simulink model "AircraftGainScheduling"  (R2022a)
settings: Solver=VariableStepAuto  StartTime=0.0  StopTime=100  RelTol=1e-3
values from neighbouring files (symbols this model uses):
  Amd = (eye(9)+Ts*Am)    [ControlMinimal.m]    (also in ExtendedControl.m; newSys.m)
  Bmd = Ts*Bm    [ControlMinimal.m]    (also in ExtendedControl.m; newSys.m)
  Cm = eye(9)    [newSys.m]
  Cmd = Cm    [ControlMinimal.m]    (also in ExtendedControl.m; newSys.m)
  Kmd = dlqr(Amd,Bmd,Q,R)    [ControlMinimal.m]    (also in ExtendedControl.m; newSys.m = lqr(Am-Ld*Cmd,Bm,Q,R))
  pointOfEquilibrium = PointOfEquilibrium(operationStates, operatingInputs )    [ControllerAroundPointOfOperation.m]    (also in InitializeAircraftPlacePolesCalculateN.m = PointOfEquilibrium([u0;v0;w0;0;0;0;0;Theta0;Psi0;0;0;100].',; TestMergeFinalLoad.m = PointOfEquilibrium(states,inputs,[-1,-1,-1]); extindere_stari_cu_perturbatie.m = PointOfEquilibrium([u0;0;w0;0;0;0;0;Theta0;Psi0;0;0;100].', ; newSys.m = PointOfEquilibrium(operationStates.', operatingInputs ))
  Ts = 0.1    [ControlMinimal.m]    (also in EstimareIntrareNecunoscuta.m; ExtendedControl.m; KalmanFilterForExtendedLinearSystem.m; LoadmUltiplePoint.m)
libraries: sharedtransform x2
settings Model: Creator=Bogdan  LastModifiedBy=Bogdan

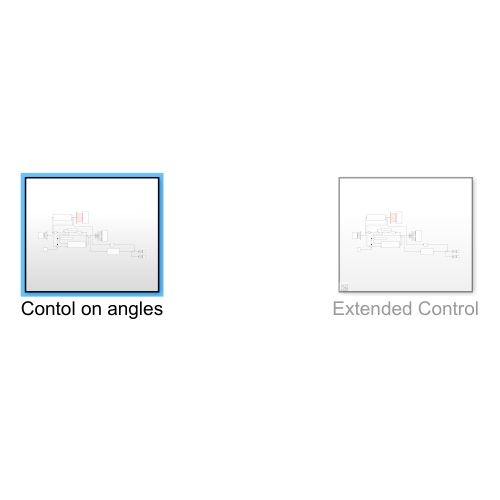
[thumbnail: Simulink's stored preview of the top-level diagram]
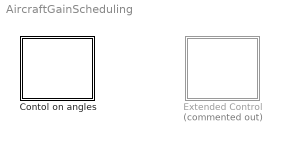
== system AircraftGainScheduling ==
  Contol on angles : Subsystem
  Extended Control : Subsystem  Commented=on

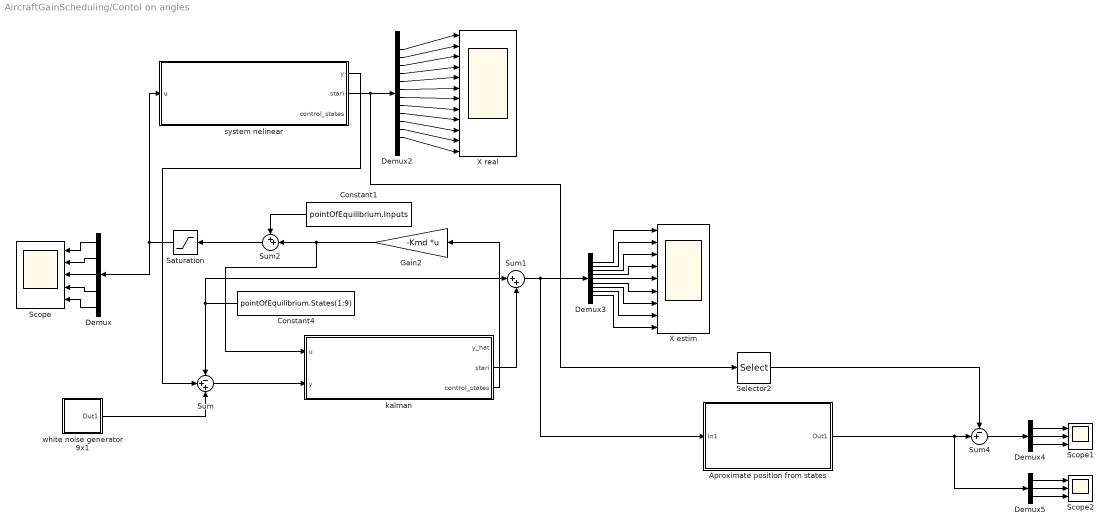
== system AircraftGainScheduling/Contol on angles ==
  Aproximate position from states : Subsystem
  Constant1 : Constant  Value=pointOfEquilibrium.Inputs
  Constant4 : Constant  Value=pointOfEquilibrium.States(1:9)
  Demux : Demux  Outputs=5
  Demux2 : Demux  Outputs=12
  Demux3 : Demux  Outputs=9
  Demux4 : Demux  Outputs=3
  Demux5 : Demux  Outputs=3
  Gain2 : Gain  Gain=-Kmd  Multiplication=Matrix(K*u) (u vector)
  Saturation : Saturate  UpperLimit=[10,pi/6,pi/6,pi/6,pi/6]  LowerLimit=[0,-pi/6,-pi/6,-pi/6,-pi/6]
  Scope : Scope  NumInputPorts=5
  Scope1 : Scope  NumInputPorts=3
  Scope2 : Scope  NumInputPorts=3
  Selector2 : Selector  InputPortWidth=12  IndexOptions=Index vector (dialog)  Indices=[10:12]  OutputSizes=1
  Sum : Sum  Inputs=-++
  Sum1 : Sum  Inputs=|++
  Sum2 : Sum  Inputs=++|
  Sum4 : Sum  Inputs=-+|
  X estim : Scope  NumInputPorts=9
  X real : Scope  NumInputPorts=12
  kalman : Subsystem
  system nelinear : Subsystem
  white noise generator 9x1 : Subsystem
  wires:
  Demux5/2 -> Scope2/2
  Demux/2 -> Scope/2
  Demux2/2 -> X real/2
  Demux3/1 -> X estim/1
  Demux5/3 -> Scope2/3
  system nelinear/2(stari) -> Selector2/1, Demux2/1
  Demux4/2 -> Scope1/2
  Constant4/1 -> Sum1/1, Sum/1
  Demux2/1 -> X real/1
  Demux3/7 -> X estim/7
  Aproximate position from states/1(Out1) -> Demux5/1, Sum4/2
  Demux/1 -> Scope/1
  Demux2/8 -> X real/8
  Demux/3 -> Scope/3
  Demux2/5 -> X real/5
  Demux4/1 -> Scope1/1
  Demux/4 -> Scope/4
  Saturation/1 -> system nelinear/1(u), Demux/1
  kalman/3(control_states) -> Gain2/1
  Demux3/5 -> X estim/5
  Sum2/1 -> Saturation/1
  Demux3/6 -> X estim/6
  Demux2/3 -> X real/3
  Sum/1 -> kalman/2(y)
  Sum1/1 -> Aproximate position from states/1(In1), Demux3/1
  Demux3/8 -> X estim/8
  Demux2/6 -> X real/6
  Sum4/1 -> Demux4/1
  Demux3/4 -> X estim/4
  white noise generator 9x1/1(Out1) -> Sum/3
  Demux5/1 -> Scope2/1
  Demux2/7 -> X real/7
  Demux4/3 -> Scope1/3
  Selector2/1 -> Sum4/1
  Demux3/9 -> X estim/9
  Demux2/11 -> X real/11
  Constant1/1 -> Sum2/1
  Demux2/12 -> X real/12
  Demux2/10 -> X real/10
  kalman/2(stari) -> Sum1/2
  Gain2/1 -> Sum2/2, kalman/1(u)
  Demux3/3 -> X estim/3
  Demux2/4 -> X real/4
  Demux3/2 -> X estim/2
  Demux/5 -> Scope/5
  Demux2/9 -> X real/9
  system nelinear/1(y) -> Sum/2

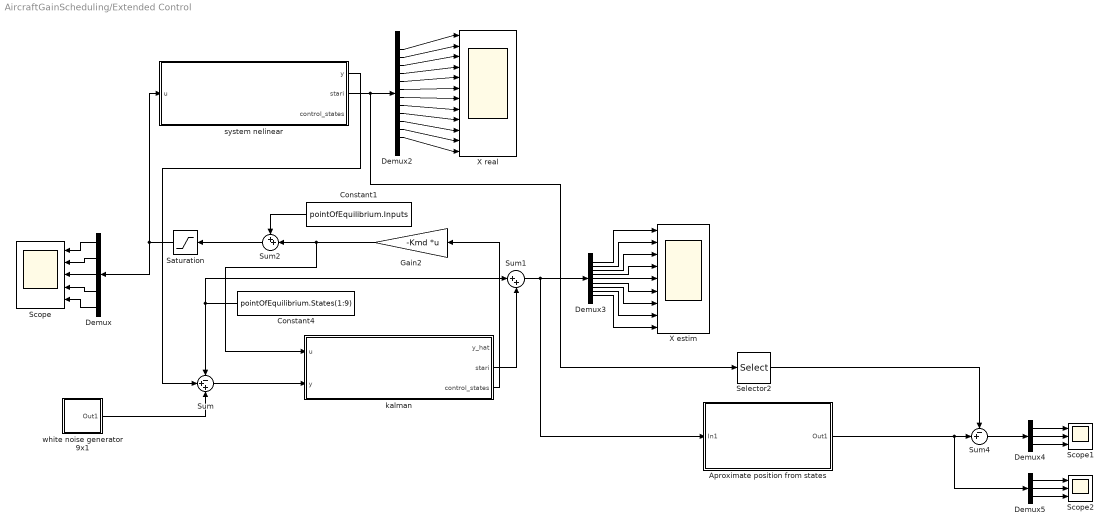
== system AircraftGainScheduling/Extended Control ==
  Aproximate position from states : Subsystem
  Constant1 : Constant  Value=pointOfEquilibrium.Inputs
  Constant4 : Constant  Value=pointOfEquilibrium.States(1:9)
  Demux : Demux  Outputs=5
  Demux2 : Demux  Outputs=12
  Demux3 : Demux  Outputs=9
  Demux4 : Demux  Outputs=3
  Demux5 : Demux  Outputs=3
  Gain2 : Gain  Gain=-Kmd  Multiplication=Matrix(K*u) (u vector)
  Saturation : Saturate  UpperLimit=[10,pi/6,pi/6,pi/6,pi/6]  LowerLimit=[0,-pi/6,-pi/6,-pi/6,-pi/6]
  Scope : Scope  NumInputPorts=5
  Scope1 : Scope  NumInputPorts=3
  Scope2 : Scope  NumInputPorts=3
  Selector2 : Selector  InputPortWidth=12  IndexOptions=Index vector (dialog)  Indices=[10:12]  OutputSizes=1
  Sum : Sum  Inputs=-++
  Sum1 : Sum  Inputs=|++
  Sum2 : Sum  Inputs=++|
  Sum4 : Sum  Inputs=-+|
  X estim : Scope  NumInputPorts=9
  X real : Scope  NumInputPorts=12
  kalman : Subsystem
  system nelinear : Subsystem
  white noise generator 9x1 : Subsystem
  wires:
  Demux5/2 -> Scope2/2
  Demux/2 -> Scope/2
  Demux2/2 -> X real/2
  Demux3/1 -> X estim/1
  Demux5/3 -> Scope2/3
  system nelinear/2(stari) -> Selector2/1, Demux2/1
  Demux4/2 -> Scope1/2
  Constant4/1 -> Sum1/1, Sum/1
  Demux2/1 -> X real/1
  Demux3/7 -> X estim/7
  Aproximate position from states/1(Out1) -> Demux5/1, Sum4/2
  Demux/1 -> Scope/1
  Demux2/8 -> X real/8
  Demux/3 -> Scope/3
  Demux2/5 -> X real/5
  Demux4/1 -> Scope1/1
  Demux/4 -> Scope/4
  Saturation/1 -> system nelinear/1(u), Demux/1
  kalman/3(control_states) -> Gain2/1
  Demux3/5 -> X estim/5
  Sum2/1 -> Saturation/1
  Demux3/6 -> X estim/6
  Demux2/3 -> X real/3
  Sum/1 -> kalman/2(y)
  Sum1/1 -> Aproximate position from states/1(In1), Demux3/1
  Demux3/8 -> X estim/8
  Demux2/6 -> X real/6
  Sum4/1 -> Demux4/1
  Demux3/4 -> X estim/4
  white noise generator 9x1/1(Out1) -> Sum/3
  Demux5/1 -> Scope2/1
  Demux2/7 -> X real/7
  Demux4/3 -> Scope1/3
  Selector2/1 -> Sum4/1
  Demux3/9 -> X estim/9
  Demux2/11 -> X real/11
  Constant1/1 -> Sum2/1
  Demux2/12 -> X real/12
  Demux2/10 -> X real/10
  kalman/2(stari) -> Sum1/2
  Gain2/1 -> Sum2/2, kalman/1(u)
  Demux3/3 -> X estim/3
  Demux2/4 -> X real/4
  Demux3/2 -> X estim/2
  Demux/5 -> Scope/5
  Demux2/9 -> X real/9
  system nelinear/1(y) -> Sum/2

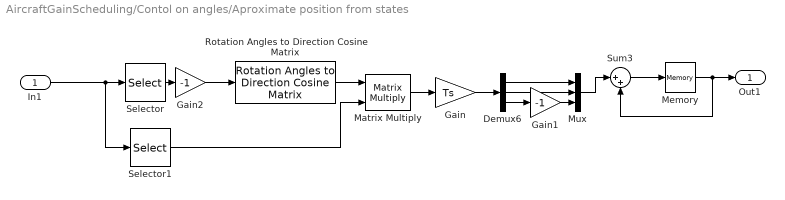
== system AircraftGainScheduling/Contol on angles/Aproximate position from states ==
  In1 : Inport
  Demux6 : Demux  Outputs=3
  Gain : Gain  Gain=Ts
  Gain1 : Gain  Gain=-1
  Gain2 : Gain  Gain=-1
  Matrix Multiply : Product  Multiplication=Matrix(*)
  Memory : Memory  InitialCondition=[0,0,100].'
  Mux : Mux  Inputs=3
  Rotation Angles to Direction Cosine Matrix : sharedtransform/Rotation Angles to Direction Cosine Matrix  rotationOrder=ZYX  aMode=aMode
      settings: SourceProductBaseCode=AE,PW,DR,MT,VE
  Selector : Selector  InputPortWidth=9  IndexOptions=Index vector (dialog)  Indices=[7:9]  OutputSizes=1
  Selector1 : Selector  InputPortWidth=9  IndexOptions=Index vector (dialog)  Indices=[1:3]  OutputSizes=1
  Sum3 : Sum  Inputs=|++
  Out1 : Outport
  wires:
  Rotation Angles to Direction Cosine Matrix/1 -> Matrix Multiply/1
  Sum3/1 -> Memory/1
  Matrix Multiply/1 -> Gain/1
  Gain/1 -> Demux6/1
  Selector1/1 -> Matrix Multiply/2
  In1/1 -> Selector1/1, Selector/1
  Demux6/2 -> Mux/2
  Mux/1 -> Sum3/1
  Demux6/1 -> Mux/1
  Memory/1 -> Sum3/2, Out1/1
  Selector/1 -> Gain2/1
  Gain2/1 -> Rotation Angles to Direction Cosine Matrix/1
  Demux6/3 -> Gain1/1
  Gain1/1 -> Mux/3

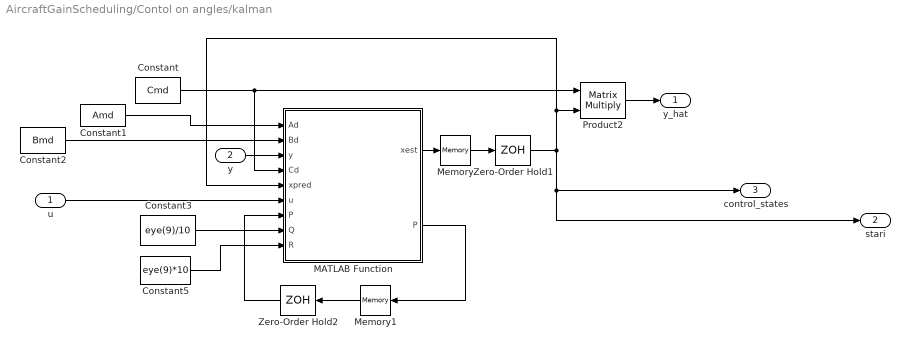
== system AircraftGainScheduling/Contol on angles/kalman ==
  u : Inport
  y : Inport  Port=2
  Constant : Constant  Value=Cmd
  Constant1 : Constant  Value=Amd
  Constant2 : Constant  Value=Bmd
  Constant3 : Constant  Value=eye(9)/10
  Constant5 : Constant  Value=eye(9)*10
  MATLAB Function : MATLAB Function  TreatAsAtomicUnit=on
  Memory : Memory  InitialCondition=zeros(9,1)
  Memory1 : Memory  InitialCondition=eye(9)*10
  Product2 : Product  Multiplication=Matrix(*)
  Zero-Order Hold1 : ZeroOrderHold  SampleTime=Ts
  Zero-Order Hold2 : ZeroOrderHold  SampleTime=Ts
  y_hat : Outport
  stari : Outport  Port=2
  control_states : Outport  Port=3
  wires:
  Constant/1 -> Product2/1, MATLAB Function/4(Cd)
  Product2/1 -> y_hat/1
  MATLAB Function/1(xest) -> Memory/1
  Memory/1 -> Zero-Order Hold1/1
  Zero-Order Hold1/1 -> control_states/1, stari/1, MATLAB Function/5(xpred), Product2/2
  y/1 -> MATLAB Function/3(y)
  u/1 -> MATLAB Function/6(u)
  Memory1/1 -> Zero-Order Hold2/1
  MATLAB Function/2(P) -> Memory1/1
  Zero-Order Hold2/1 -> MATLAB Function/7("P ")
  Constant1/1 -> MATLAB Function/1(Ad)
  Constant2/1 -> MATLAB Function/2(Bd)
  Constant3/1 -> MATLAB Function/8(Q)
  Constant5/1 -> MATLAB Function/9(R)

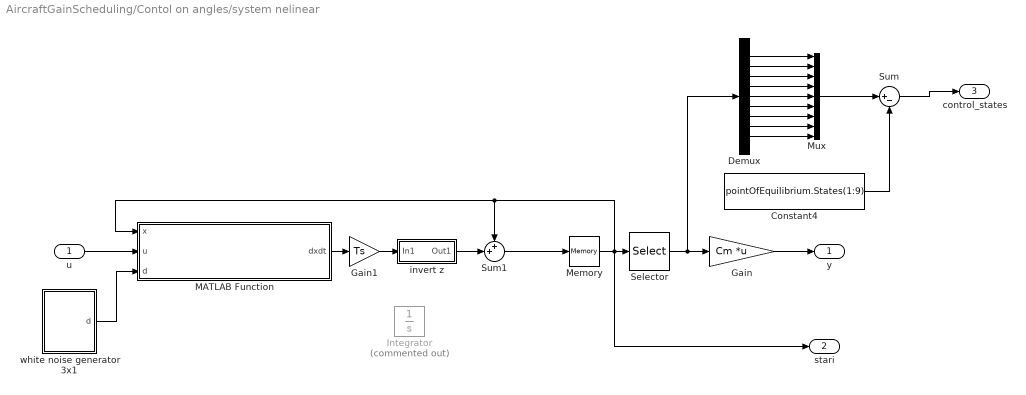
== system AircraftGainScheduling/Contol on angles/system nelinear ==
  u : Inport
  Constant4 : Constant  Value=pointOfEquilibrium.States(1:9)
  Demux : Demux  Outputs=9
  Gain : Gain  Gain=Cm  Multiplication=Matrix(K*u) (u vector)
  Gain1 : Gain  Gain=Ts
  Integrator : Integrator  Commented=on  InitialCondition=pointOfEquilibrium.States.'
  MATLAB Function : MATLAB Function  TreatAsAtomicUnit=on
  Memory : Memory  InitialCondition=pointOfEquilibrium.States.'+[1,1,1,0,0,0,0,0,0,0,0,0].'
  Mux : Mux  Inputs=9
  Selector : Selector  InputPortWidth=12  IndexOptions=Index vector (dialog)  Indices=[1:9]  OutputSizes=1
  Sum : Sum  Inputs=|+-
  Sum1 : Sum  Inputs=++|
  invert z : Subsystem
  white noise generator 3x1 : Subsystem
  y : Outport
  stari : Outport  Port=2
  control_states : Outport  Port=3
  wires:
  Gain/1 -> y/1
  Demux/2 -> Mux/2
  Demux/5 -> Mux/5
  Demux/3 -> Mux/3
  Demux/6 -> Mux/6
  Demux/4 -> Mux/4
  Demux/1 -> Mux/1
  Demux/7 -> Mux/7
  Demux/8 -> Mux/8
  Demux/9 -> Mux/9
  Selector/1 -> Gain/1, Demux/1
  u/1 -> MATLAB Function/2(u)
  Mux/1 -> Sum/1
  Sum/1 -> control_states/1
  Constant4/1 -> Sum/2
  white noise generator 3x1/1(d) -> MATLAB Function/3(d)
  Memory/1 -> stari/1, MATLAB Function/1(x), Sum1/1, Selector/1
  MATLAB Function/1(dxdt) -> Gain1/1
  Sum1/1 -> Memory/1
  Gain1/1 -> invert z/1(In1)
  invert z/1(Out1) -> Sum1/2

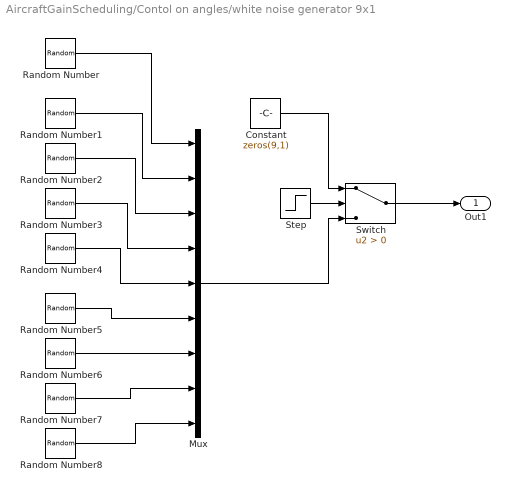
== system AircraftGainScheduling/Contol on angles/white noise generator 9x1 ==
  Constant : Constant  Value=zeros(9,1)
  Mux : Mux  Inputs=9
  Random Number : RandomNumber  Variance=.5  SampleTime=Ts
  Random Number1 : RandomNumber  Variance=.5  SampleTime=Ts
  Random Number2 : RandomNumber  Variance=.5  SampleTime=Ts
  Random Number3 : RandomNumber  Variance=.03  SampleTime=Ts
  Random Number4 : RandomNumber  Variance=.03  SampleTime=Ts
  Random Number5 : RandomNumber  Variance=.03  SampleTime=Ts
  Random Number6 : RandomNumber  Variance=.05  SampleTime=Ts
  Random Number7 : RandomNumber  Variance=.05  SampleTime=Ts
  Random Number8 : RandomNumber  Variance=.05  SampleTime=Ts
  Step : Step  Time=5  SampleTime=0
  Switch : Switch  Criteria=u2 > Threshold  SaturateOnIntegerOverflow=off  InputSameDT=off
  Out1 : Outport
  wires:
  Random Number7/1 -> Mux/8
  Random Number3/1 -> Mux/4
  Random Number4/1 -> Mux/5
  Random Number2/1 -> Mux/3
  Random Number5/1 -> Mux/6
  Random Number8/1 -> Mux/9
  Random Number6/1 -> Mux/7
  Random Number1/1 -> Mux/2
  Random Number/1 -> Mux/1
  Step/1 -> Switch/2
  Switch/1 -> Out1/1
  Mux/1 -> Switch/3
  Constant/1 -> Switch/1

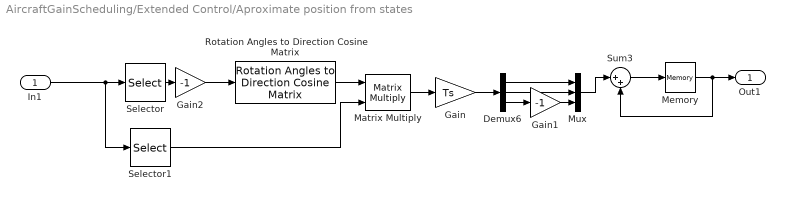
== system AircraftGainScheduling/Extended Control/Aproximate position from states ==
  In1 : Inport
  Demux6 : Demux  Outputs=3
  Gain : Gain  Gain=Ts
  Gain1 : Gain  Gain=-1
  Gain2 : Gain  Gain=-1
  Matrix Multiply : Product  Multiplication=Matrix(*)
  Memory : Memory  InitialCondition=[0,0,100].'
  Mux : Mux  Inputs=3
  Rotation Angles to Direction Cosine Matrix : sharedtransform/Rotation Angles to Direction Cosine Matrix  rotationOrder=ZYX  aMode=aMode
      settings: SourceProductBaseCode=AE,PW,DR,MT,VE
  Selector : Selector  InputPortWidth=9  IndexOptions=Index vector (dialog)  Indices=[7:9]  OutputSizes=1
  Selector1 : Selector  InputPortWidth=9  IndexOptions=Index vector (dialog)  Indices=[1:3]  OutputSizes=1
  Sum3 : Sum  Inputs=|++
  Out1 : Outport
  wires:
  Rotation Angles to Direction Cosine Matrix/1 -> Matrix Multiply/1
  Sum3/1 -> Memory/1
  Matrix Multiply/1 -> Gain/1
  Gain/1 -> Demux6/1
  Selector1/1 -> Matrix Multiply/2
  In1/1 -> Selector1/1, Selector/1
  Demux6/2 -> Mux/2
  Mux/1 -> Sum3/1
  Demux6/1 -> Mux/1
  Memory/1 -> Sum3/2, Out1/1
  Selector/1 -> Gain2/1
  Gain2/1 -> Rotation Angles to Direction Cosine Matrix/1
  Demux6/3 -> Gain1/1
  Gain1/1 -> Mux/3

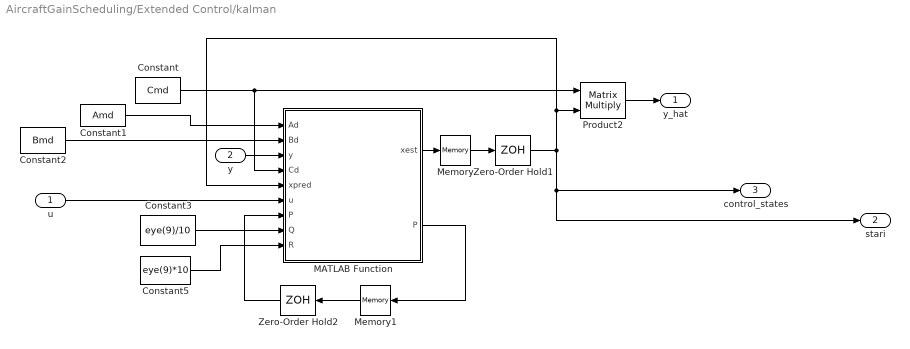
== system AircraftGainScheduling/Extended Control/kalman ==
  u : Inport
  y : Inport  Port=2
  Constant : Constant  Value=Cmd
  Constant1 : Constant  Value=Amd
  Constant2 : Constant  Value=Bmd
  Constant3 : Constant  Value=eye(9)/10
  Constant5 : Constant  Value=eye(9)*10
  MATLAB Function : MATLAB Function  TreatAsAtomicUnit=on
  Memory : Memory  InitialCondition=zeros(9,1)
  Memory1 : Memory  InitialCondition=eye(9)*10
  Product2 : Product  Multiplication=Matrix(*)
  Zero-Order Hold1 : ZeroOrderHold  SampleTime=Ts
  Zero-Order Hold2 : ZeroOrderHold  SampleTime=Ts
  y_hat : Outport
  stari : Outport  Port=2
  control_states : Outport  Port=3
  wires:
  Constant/1 -> Product2/1, MATLAB Function/4(Cd)
  Product2/1 -> y_hat/1
  MATLAB Function/1(xest) -> Memory/1
  Memory/1 -> Zero-Order Hold1/1
  Zero-Order Hold1/1 -> control_states/1, stari/1, MATLAB Function/5(xpred), Product2/2
  y/1 -> MATLAB Function/3(y)
  u/1 -> MATLAB Function/6(u)
  Memory1/1 -> Zero-Order Hold2/1
  MATLAB Function/2(P) -> Memory1/1
  Zero-Order Hold2/1 -> MATLAB Function/7("P ")
  Constant1/1 -> MATLAB Function/1(Ad)
  Constant2/1 -> MATLAB Function/2(Bd)
  Constant3/1 -> MATLAB Function/8(Q)
  Constant5/1 -> MATLAB Function/9(R)

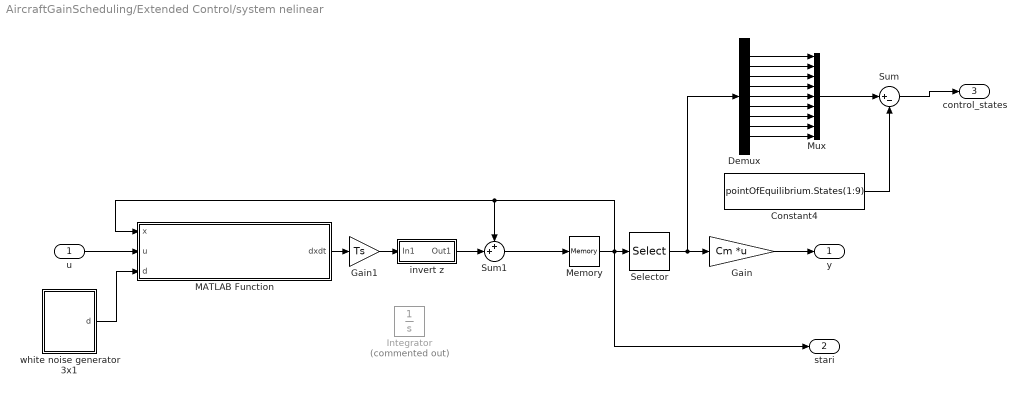
== system AircraftGainScheduling/Extended Control/system nelinear ==
  u : Inport
  Constant4 : Constant  Value=pointOfEquilibrium.States(1:9)
  Demux : Demux  Outputs=9
  Gain : Gain  Gain=Cm  Multiplication=Matrix(K*u) (u vector)
  Gain1 : Gain  Gain=Ts
  Integrator : Integrator  Commented=on  InitialCondition=pointOfEquilibrium.States.'
  MATLAB Function : MATLAB Function  TreatAsAtomicUnit=on
  Memory : Memory  InitialCondition=pointOfEquilibrium.States.'+[1,1,1,0,0,0,0,0,0,0,0,0].'
  Mux : Mux  Inputs=9
  Selector : Selector  InputPortWidth=12  IndexOptions=Index vector (dialog)  Indices=[1:9]  OutputSizes=1
  Sum : Sum  Inputs=|+-
  Sum1 : Sum  Inputs=++|
  invert z : Subsystem
  white noise generator 3x1 : Subsystem
  y : Outport
  stari : Outport  Port=2
  control_states : Outport  Port=3
  wires:
  Gain/1 -> y/1
  Demux/2 -> Mux/2
  Demux/5 -> Mux/5
  Demux/3 -> Mux/3
  Demux/6 -> Mux/6
  Demux/4 -> Mux/4
  Demux/1 -> Mux/1
  Demux/7 -> Mux/7
  Demux/8 -> Mux/8
  Demux/9 -> Mux/9
  Selector/1 -> Gain/1, Demux/1
  u/1 -> MATLAB Function/2(u)
  Mux/1 -> Sum/1
  Sum/1 -> control_states/1
  Constant4/1 -> Sum/2
  white noise generator 3x1/1(d) -> MATLAB Function/3(d)
  Memory/1 -> stari/1, MATLAB Function/1(x), Sum1/1, Selector/1
  MATLAB Function/1(dxdt) -> Gain1/1
  Sum1/1 -> Memory/1
  Gain1/1 -> invert z/1(In1)
  invert z/1(Out1) -> Sum1/2

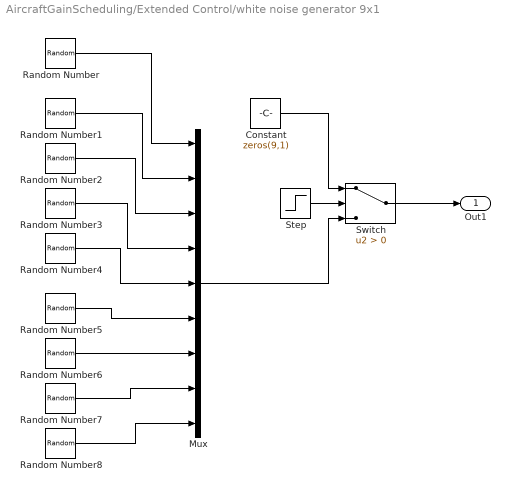
== system AircraftGainScheduling/Extended Control/white noise generator 9x1 ==
  Constant : Constant  Value=zeros(9,1)
  Mux : Mux  Inputs=9
  Random Number : RandomNumber  Variance=.5  SampleTime=Ts
  Random Number1 : RandomNumber  Variance=.5  SampleTime=Ts
  Random Number2 : RandomNumber  Variance=.5  SampleTime=Ts
  Random Number3 : RandomNumber  Variance=.03  SampleTime=Ts
  Random Number4 : RandomNumber  Variance=.03  SampleTime=Ts
  Random Number5 : RandomNumber  Variance=.03  SampleTime=Ts
  Random Number6 : RandomNumber  Variance=.05  SampleTime=Ts
  Random Number7 : RandomNumber  Variance=.05  SampleTime=Ts
  Random Number8 : RandomNumber  Variance=.05  SampleTime=Ts
  Step : Step  Time=5  SampleTime=0
  Switch : Switch  Criteria=u2 > Threshold  SaturateOnIntegerOverflow=off  InputSameDT=off
  Out1 : Outport
  wires:
  Random Number7/1 -> Mux/8
  Random Number3/1 -> Mux/4
  Random Number4/1 -> Mux/5
  Random Number2/1 -> Mux/3
  Random Number5/1 -> Mux/6
  Random Number8/1 -> Mux/9
  Random Number6/1 -> Mux/7
  Random Number1/1 -> Mux/2
  Random Number/1 -> Mux/1
  Step/1 -> Switch/2
  Switch/1 -> Out1/1
  Mux/1 -> Switch/3
  Constant/1 -> Switch/1

== system AircraftGainScheduling/Contol on angles/system nelinear/invert z ==
  In1 : Inport
  Demux1 : Demux  Outputs=12
  Gain2 : Gain  Gain=-1
  Mux1 : Mux  Inputs=12
  Out1 : Outport
  wires:
  Demux1/3 -> Mux1/3
  Demux1/9 -> Mux1/9
  Demux1/6 -> Mux1/6
  Demux1/2 -> Mux1/2
  Demux1/11 -> Mux1/11
  Demux1/8 -> Mux1/8
  In1/1 -> Demux1/1
  Demux1/4 -> Mux1/4
  Gain2/1 -> Mux1/12
  Demux1/10 -> Mux1/10
  Demux1/12 -> Gain2/1
  Demux1/5 -> Mux1/5
  Demux1/7 -> Mux1/7
  Demux1/1 -> Mux1/1
  Mux1/1 -> Out1/1

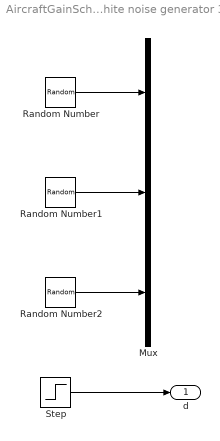
== system AircraftGainScheduling/Contol on angles/system nelinear/white noise generator 3x1 ==
  Mux : Mux  Inputs=3
  Random Number : RandomNumber  Variance=.3  SampleTime=Ts
  Random Number1 : RandomNumber  Variance=.1  SampleTime=Ts
  Random Number2 : RandomNumber  Variance=.1  SampleTime=Ts
  Step : Step  Time=0  Before=[0,0,0]  After=[1,1,1]  SampleTime=0
  d : Outport
  wires:
  Random Number2/1 -> Mux/3
  Random Number1/1 -> Mux/2
  Random Number/1 -> Mux/1
  Step/1 -> d/1

== system AircraftGainScheduling/Extended Control/system nelinear/invert z ==
  In1 : Inport
  Demux1 : Demux  Outputs=12
  Gain2 : Gain  Gain=-1
  Mux1 : Mux  Inputs=12
  Out1 : Outport
  wires:
  Demux1/3 -> Mux1/3
  Demux1/9 -> Mux1/9
  Demux1/6 -> Mux1/6
  Demux1/2 -> Mux1/2
  Demux1/11 -> Mux1/11
  Demux1/8 -> Mux1/8
  In1/1 -> Demux1/1
  Demux1/4 -> Mux1/4
  Gain2/1 -> Mux1/12
  Demux1/10 -> Mux1/10
  Demux1/12 -> Gain2/1
  Demux1/5 -> Mux1/5
  Demux1/7 -> Mux1/7
  Demux1/1 -> Mux1/1
  Mux1/1 -> Out1/1

== system AircraftGainScheduling/Extended Control/system nelinear/white noise generator 3x1 ==
  Mux : Mux  Inputs=3
  Random Number : RandomNumber  Variance=.3  SampleTime=Ts
  Random Number1 : RandomNumber  Variance=.1  SampleTime=Ts
  Random Number2 : RandomNumber  Variance=.1  SampleTime=Ts
  Step : Step  Time=50  Before=[0,0,0]  After=[1,0,0]  SampleTime=0
  d : Outport
  wires:
  Random Number2/1 -> Mux/3
  Random Number1/1 -> Mux/2
  Random Number/1 -> Mux/1
  Step/1 -> d/1

== matlab function AircraftGainScheduling/Extended Control/kalman/MATLAB Function ==
  data: Ad input; Bd input; xest output; y input; Cd input; xpred input; u input; P input; P output; Q input; R input
function [xest,P] = KalmanFilterNoCap(Ad, Bd, y, Cd, xpred, u, P, Q, R)
    xpred=Ad*xpred+Bd*u;
    Pred=Ad*P*Ad.'+Q;
    Kn=Pred*Cd.'/(Cd*Pred*Cd.'+R);
    xest=xpred+Kn*(y-Cd*xpred);
    P=(eye(9)-Kn*Cd)*Pred*(eye(9)-Kn*Cd).'+Kn*R*Kn.';
end

== matlab function AircraftGainScheduling/Extended Control/system nelinear/MATLAB Function ==
  data: x input; u input; dxdt output; d input
function dxdt = aircraftSystem(x,u,d)
obj=aircraft();
g=9.81;
%take inputs from vector
T=u(1);
DeltaSt=getAngle(u(2));
DeltaRud=getAngle(u(3));
DeltaAlL=getAngle(u(4));
DeltaAlR=getAngle(u(5));
%take states from vector
u=x(1)-d(1); 
v=x(2)-d(2);
w=x(3)-d(3);
p=x(4);
q=x(5);
r=x(6);
Phi=getAngle(x(7));
Theta=getAngle(x(8));
Psi=getAngle(x(9));
px=x(10);
py=x(11);
pz=x(12);
%vant in earth system
R=Rearth2body(Phi,Theta,Psi);
d=R*d;


alpha=atan2(w,u);
beta=atan2(v,u);
Va2=(u)^2+(v)^2+(w)^2;
Cdw=0.0115*alpha*180/pi+1;
Cdfus=0.075*alpha*180/pi+1;
CyFus=0.075*beta*180/pi;
Cyrud=0.075*(beta+DeltaRud)*180/pi;
Clw=0.11*alpha*180/pi;
ClSt=0.11*(alpha+DeltaSt)*180/pi;
ClwL=0.11*(DeltaAlL+alpha)*180/pi;
ClwR=0.11*(DeltaAlR+alpha)*180/pi;
G=[0;0;obj.m*g];
Fa=[-(Cdw*obj.Af_wing+Cdfus*obj.Af_fuselage)*obj.ro*Va2/2;
-(CyFus*obj.Alat+Cyrud*obj.Arudder)*obj.ro*Va2/2;
-(Clw*obj.Aw+ClSt*obj.Ast+ClwL*obj.Aaileron/2+ClwR*obj.Aaileron/2)*obj.ro*Va2/2];
l_fus=0.01;
Ft=[T;0;0];
% fara vant alpha=theta
% beta=psi
F=Ft+Rearth2body(0,Theta,Psi)*Fa+R*G;

L_bar=obj.l3*obj.Aaileron*(ClwL-ClwR)*obj.ro*Va2/2;
M=(obj.l1*Clw*obj.Aw+ClSt*obj.l2*obj.Ast)*obj.ro*Va2/2;
N=(obj.l2*Cyrud*obj.Arudder+CyFus*l_fus*obj.Alat)*obj.ro*Va2/2;

Moments=[L_bar;M;N];
dxdt=[F/obj.m-cross([p;q;r],[u;v;w]);
    obj.Iinv*(Moments-cross([p;q;r],obj.I*[p;q;r]));
    H(Phi,Theta)*[p;q;r];
    Rbody2earth(-Phi,-Theta,-Psi)*[u;v;w]];
end

== matlab function AircraftGainScheduling/Contol on angles/system nelinear/MATLAB Function ==
  data: x input; u input; dxdt output; d input
function dxdt = aircraftSystem(x,u,d)
obj=aircraft();
g=9.81;
%take inputs from vector
T=u(1);
DeltaSt=getAngle(u(2));
DeltaRud=getAngle(u(3));
DeltaAlL=getAngle(u(4));
DeltaAlR=getAngle(u(5));
%take states from vector
u=x(1)-d(1); 
v=x(2)-d(2);
w=x(3)-d(3);
p=x(4);
q=x(5);
r=x(6);
Phi=getAngle(x(7));
Theta=getAngle(x(8));
Psi=getAngle(x(9));
px=x(10);
py=x(11);
pz=x(12);
%vant in earth system
R=Rearth2body(Phi,Theta,Psi);
d=R*d;


alpha=atan2(w,u);
beta=atan2(v,u);
Va2=(u)^2+(v)^2+(w)^2;
Cdw=0.0115*alpha*180/pi+1;
Cdfus=0.075*alpha*180/pi+1;
CyFus=0.075*beta*180/pi;
Cyrud=0.075*(beta+DeltaRud)*180/pi;
Clw=0.11*alpha*180/pi;
ClSt=0.11*(alpha+DeltaSt)*180/pi;
ClwL=0.11*(DeltaAlL+alpha)*180/pi;
ClwR=0.11*(DeltaAlR+alpha)*180/pi;
G=[0;0;obj.m*g];
Fa=[-(Cdw*obj.Af_wing+Cdfus*obj.Af_fuselage)*obj.ro*Va2/2;
-(CyFus*obj.Alat+Cyrud*obj.Arudder)*obj.ro*Va2/2;
-(Clw*obj.Aw+ClSt*obj.Ast+ClwL*obj.Aaileron/2+ClwR*obj.Aaileron/2)*obj.ro*Va2/2];
l_fus=0.01;
Ft=[T;0;0];
% fara vant alpha=theta
% beta=psi
F=Ft+Rearth2body(0,Theta,Psi)*Fa+R*G;

L_bar=obj.l3*obj.Aaileron*(ClwL-ClwR)*obj.ro*Va2/2;
M=(obj.l1*Clw*obj.Aw+ClSt*obj.l2*obj.Ast)*obj.ro*Va2/2;
N=(obj.l2*Cyrud*obj.Arudder+CyFus*l_fus*obj.Alat)*obj.ro*Va2/2;

Moments=[L_bar;M;N];
dxdt=[F/obj.m-cross([p;q;r],[u;v;w]);
    obj.Iinv*(Moments-cross([p;q;r],obj.I*[p;q;r]));
    H(Phi,Theta)*[p;q;r];
    Rbody2earth(-Phi,-Theta,-Psi)*[u;v;w]];
end

== matlab function AircraftGainScheduling/Contol on angles/kalman/MATLAB Function ==
  data: Ad input; Bd input; xest output; y input; Cd input; xpred input; u input; P input; P output; Q input; R input
function [xest,P] = KalmanFilterNoCap(Ad, Bd, y, Cd, xpred, u, P, Q, R)
    xpred=Ad*xpred+Bd*u;
    Pred=Ad*P*Ad.'+Q;
    Kn=Pred*Cd.'/(Cd*Pred*Cd.'+R);
    xest=xpred+Kn*(y-Cd*xpred);
    P=(eye(9)-Kn*Cd)*Pred*(eye(9)-Kn*Cd).'+Kn*R*Kn.';
end
